simulink model "first_model"  (R2020b)
settings: Solver=VariableStepAuto  StartTime=0.0  StopTime=10.0  RelTol=1e-3
settings Model: Creator=SWARUP  LastModifiedBy=SWARUP

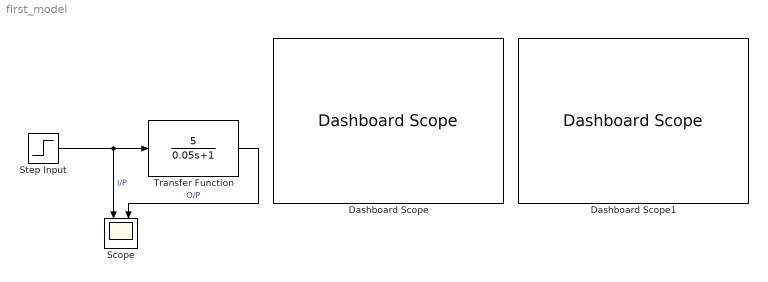
== system first_model ==
  Dashboard Scope : DashboardScope
  Dashboard Scope1 : DashboardScope
  "Scope " : Scope  NumInputPorts=2
  Step Input : Step  Before=1  After=5  SampleTime=0
  Transfer Function : TransferFcn  Numerator=[5]  Denominator=[0.05 1]
  wires:
  Step Input/1 -> "Scope "/1, Transfer Function/1  "I/P"
  Transfer Function/1 -> "Scope "/2  "O/P"
